simulink model "TA1415"  (R2022a)
settings: Solver=VariableStepAuto  StartTime=0.0  StopTime=69  RelTol=1e-3
model workspace (MAT data in the model file):
  KE = 0.008112779366
  XA0 = 0
  XG0 = 0.02
  XG_max = 5.46511903061
  aE = 0.150776877402
  k1 = 0.477209468937
  k2 = 0.908904061287
  k3 = 1.2417823041
  n0 = 2.86068812818
  rleak = 0.277729865506
  stepTime = 9.3050645559
settings Model: Creator=tomok  LastModifiedBy=tomok
settings DataIOCC: ReturnWorkspaceOutputsName=SDOSimTest_Log

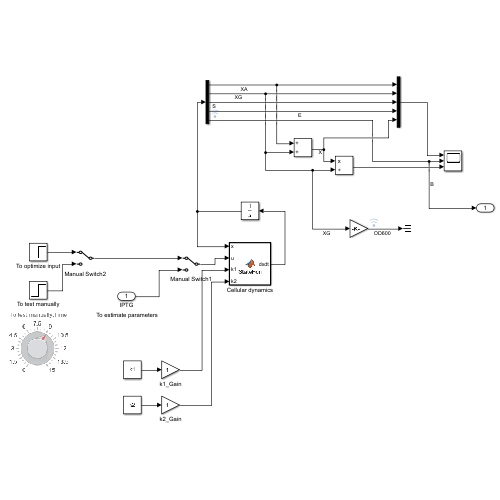
[thumbnail: Simulink's stored preview of the top-level diagram]
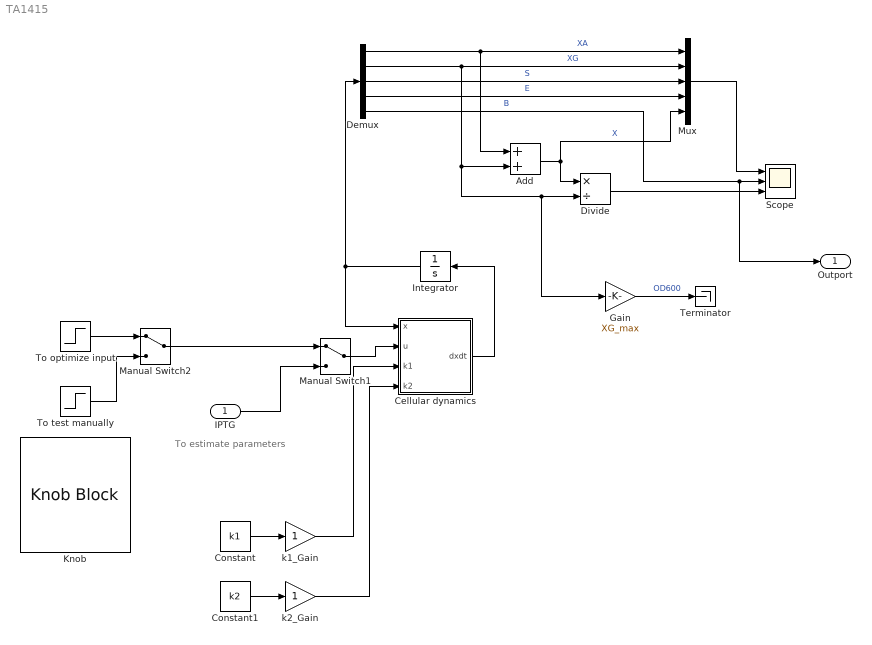
== system TA1415 ==
  note: To estimate parameters
  IPTG : Inport
  Add : Sum
  Cellular dynamics : MATLAB Function  TreatAsAtomicUnit=on
  Constant : Constant  Value=k1
  Constant1 : Constant  Value=k2
  Demux : Demux  Outputs=5
  Divide : Product  Inputs=*/
  Gain : Gain  Gain=XG_max
  Integrator : Integrator  InitialCondition=[n0*XG0; XG0; 1-n0*XG0-XG0; 0; 0]
  Knob : KnobBlock  ScaleMax=15
  Manual Switch1 : ManualSwitch
  Manual Switch2 : ManualSwitch
  Mux : Mux  Inputs=5
  Scope : Scope  NumInputPorts=3
  Terminator : Terminator
  To optimize input : Step  Time=stepTime  SampleTime=0
  To test manually : Step  Time=9  SampleTime=0
  k1_Gain : Gain
  k2_Gain : Gain
  Outport : Outport
  wires:
  Cellular dynamics/1(dxdt) -> Integrator/1
  Integrator/1 -> Demux/1, Cellular dynamics/1(x)
  Demux/1 -> Add/1, Mux/1  "XA"
  Demux/2 -> Add/2, Gain/1, Divide/2, Mux/2  "XG"
  Demux/3 -> Mux/3  "S"
  Add/1 -> Divide/1, Mux/5  "X"
  Divide/1 -> Scope/3
  Mux/1 -> Scope/1
  To test manually/1 -> Manual Switch2/2
  Demux/4 -> Mux/4  "E"
  IPTG/1 -> Manual Switch1/2
  Manual Switch1/1 -> Cellular dynamics/2(u)
  Gain/1 -> Terminator/1  "OD600"
  To optimize input/1 -> Manual Switch2/1
  Manual Switch2/1 -> Manual Switch1/1
  Constant/1 -> k1_Gain/1
  k1_Gain/1 -> Cellular dynamics/3(k1)
  k2_Gain/1 -> Cellular dynamics/4(k2)
  Constant1/1 -> k2_Gain/1
  Demux/5 -> Outport/1, Scope/2  "B"

== matlab function TA1415/Cellular dynamics ==
  data: x input; dxdt output; u input; k3 parameter; rleak parameter; aE parameter; KE parameter; k1 input; k2 input
function dxdt = StateFcn(x,u,k3, rleak, aE, KE, k1, k2)
%% Parameters
% k1 = 0.5;
% k2 = 1;
% k3 = 2;
% rleak = 0.3;
% aE = 0.3;
% KE = 0.2;

%% Input variables and feed concentration

%% State variables
XA = x(1);
XG = x(2);
S = x(3);
E = x(4);

%% reaction rates
v1 = k1*S*(XA + XG + E)*(1 - (1 - rleak)*u); % substrate uptake
v2 = k2*XA*(XG + E);       % biomass formation (growth)
v3 = k3*(E/(E + KE))*XG;

%% ODEs
dXAdt = v1 - v2;
dXGdt = v2*(1 - aE*u);
dSdt = -v1;
dEdt = v2*aE*u;
dBdt = v3;

dxdt = [dXAdt; dXGdt; dSdt; dEdt; dBdt];

% lower limit of states
dxdt(x < 0 & dxdt < 0) = 0;
end
